simulink library "fastled17b"  (R2017b)
settings: Solver=VariableStepAuto  StartTime=0.0  StopTime=10.0  RelTol=1e-3
settings Model: Creator=brianhannan  LastModifiedBy=brianhannan
settings DataIOCC: ReturnWorkspaceOutputs=on
settings SFSimCC: SimUseLocalCustomCode=on
settings RTWCC: RTWUseLocalCustomCode=on

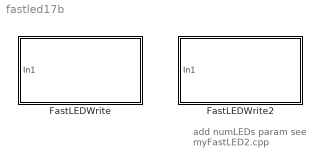
== system fastled17b ==
  note: add numLEDs param
      | see myFastLED2.cpp
  FastLEDWrite : Subsystem  mask(FastLEDWrite){pinNum=5}
      mask prompts: pinNum "Data pin:"
      mask help: Control a WS2812B LED strip using FastLED and an Arduino Uno.
      mask init:
      | % add 1 to to pinNum b/c starts at 2
      | pinNum = pinNum + 1;
      mask TypeOptions pinNum: 2 | 3 | 4 | 5 | 6 | 7 | 8 | 9 | 10 | 11 | 12 | 13
      mask Display: disp('Fast LED Write')
  FastLEDWrite2 : Subsystem  mask(FastLEDWrite){pinNum=5, numLEDs=3}
      mask prompts: pinNum "Data pin:"; numLEDs "Num. LEDs:"
      mask help: Control a WS2812B LED strip using FastLED and an Arduino Uno.
      mask init:
      | % add 1 to to pinNum b/c starts at 2
      | pinNum = pinNum + 1;
      mask TypeOptions pinNum: 2 | 3 | 4 | 5 | 6 | 7 | 8 | 9 | 10 | 11 | 12 | 13
      mask Display: disp('Fast LED Write')

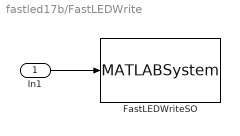
== system fastled17b/FastLEDWrite ==
  In1 : Inport
  FastLEDWriteSO : MATLABSystem  System=FastLEDWrite  Pin=pinNum
      mask Type: FastLEDWrite
      mask Display:
      | disp('FastLED Write');
      | port_label('input',1,'u');
  wires:
  In1/1 -> FastLEDWriteSO/1

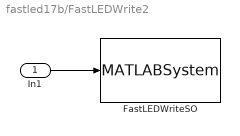
== system fastled17b/FastLEDWrite2 ==
  In1 : Inport
  FastLEDWriteSO : MATLABSystem  System=FastLEDWrite2  Pin=pinNum  NumLEDs=numLEDs
      mask Type: FastLEDWrite2
      mask Display:
      | disp('FastLED Write');
      | port_label('input',1,'u');
  wires:
  In1/1 -> FastLEDWriteSO/1
